simulink model "Simu"  (R2019a)
settings: Solver=VariableStepAuto  StartTime=0.0  StopTime=10.0  RelTol=1e-3
libraries: simulink x1
settings Model: Creator=juan.montorfano  LastModifiedBy=juan.montorfano

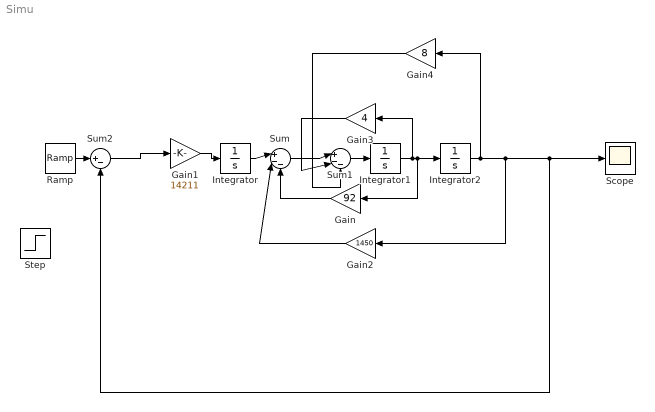
== system Simu ==
  Gain : Gain  Gain=92
  Gain1 : Gain  Gain=14211
  Gain2 : Gain  Gain=1450
  Gain3 : Gain  Gain=4
  Gain4 : Gain  Gain=8
  Integrator : Integrator
  Integrator1 : Integrator
  Integrator2 : Integrator
  Ramp : simulink/Sources/Ramp  slope=1  start=0  InitialOutput=0
  Scope : Scope
  Step : Step  Time=0  SampleTime=0
  Sum : Sum  Inputs=|+--
  Sum1 : Sum  Inputs=|+--
  Sum2 : Sum  Inputs=|+-
  wires:
  Sum2/1 -> Gain1/1
  Integrator/1 -> Sum/1
  Sum/1 -> Sum1/1
  Sum1/1 -> Integrator1/1
  Gain1/1 -> Integrator/1
  Integrator2/1 -> Gain4/1, Scope/1, Sum2/2, Gain2/1
  Gain/1 -> Sum/3
  Gain2/1 -> Sum/2
  Integrator1/1 -> Gain3/1, Gain/1, Integrator2/1
  Gain3/1 -> Sum1/2
  Gain4/1 -> Sum1/3
  Ramp/1 -> Sum2/1
